simulink model "onlyFins2Acc"  (R2015a)
settings: Solver=ode45  StartTime=0.0  StopTime=10.0  RelTol=1e-3
values from neighbouring files (symbols this model uses):
  CLd = pi*ARf*Sfins/(1+sqrt(1+(pi*ARf/(2*0.7))^2))/S    [loadModel_EB.m]
  rho = 1.21    [loadModel_EB.m]
  S = pi*D_booster^4/4    (= 0.0131916732161)    [loadModel_EB.m]
  Vx = M*sqrt(gamma_air*r*T)    [loadModel_EB.m]
undefined symbols (not defined in the file or in its folder): flexi
settings Model: Creator=anatole  LastModifiedBy=anatole

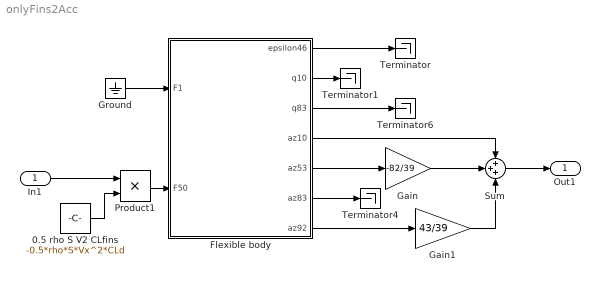
== system onlyFins2Acc ==
  In1 : Inport
  0.5 rho S V2 CLfins : Constant  Value=-0.5*rho*S*Vx^2*CLd
  Flexible body : Subsystem
      mask Display:
      | port_label('input',1,'Lateral Thrust')
      | 
      | port_label('output',1,'\epsilon_{46}','texmode','on')
      | port_label('output',2,'q_{10}','texmode','on')
      | port_label('output',3,'q_{83}','texmode','on')
      | port_label('output',4,'a_{z10}','texmode','on')
      | port_label('output',5,'a_{z53}','texmode','on')
      | port_label('output',6,'a_{z83}','texmode','on')
      | port_label('output',7,'a_{z92}','texmode','on')
  Gain : Gain  Gain=-82/39
  Gain1 : Gain  Gain=43/39
  Ground : Ground
  Product1 : Product
  Sum : Sum  Inputs=+++
  Terminator{,1,4,6} (4 alike) : Terminator
  Out1 : Outport
  wires:
  In1/1 -> Product1/1
  Product1/1 -> Flexible body/2(F50)
  0.5 rho S V2 CLfins/1 -> Product1/2
  Ground/1 -> Flexible body/1(F1)
  Flexible body/4(az10) -> Sum/1
  Flexible body/5(az53) -> Gain/1
  Flexible body/6(az83) -> Terminator4/1
  Flexible body/7(az92) -> Gain1/1
  Flexible body/1(epsilon46) -> Terminator/1
  Flexible body/2(q10) -> Terminator1/1
  Flexible body/3(q83) -> Terminator6/1
  Gain/1 -> Sum/2
  Gain1/1 -> Sum/3
  Sum/1 -> Out1/1

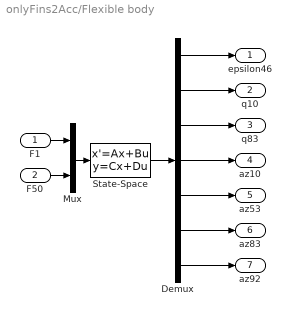
== system onlyFins2Acc/Flexible body ==
  F1 : Inport
  F50 : Inport  Port=2
  Demux : Demux  Outputs=7
  Mux : Mux  Inputs=2
  State-Space : StateSpace  A=flexi.a  B=flexi.b  C=flexi.c  D=flexi.d  X0=0
  epsilon46 : Outport
  q10 : Outport  Port=2
  q83 : Outport  Port=3
  az10 : Outport  Port=4
  az53 : Outport  Port=5
  az83 : Outport  Port=6
  az92 : Outport  Port=7
  wires:
  State-Space/1 -> Demux/1
  Demux/1 -> epsilon46/1
  Demux/2 -> q10/1
  Demux/3 -> q83/1
  Demux/4 -> az10/1
  Demux/5 -> az53/1
  Demux/6 -> az83/1
  Demux/7 -> az92/1
  Mux/1 -> State-Space/1
  F1/1 -> Mux/1
  F50/1 -> Mux/2
